simulink model "Q_2_1_4_PID_FF_Comp_Emulation_DISCRETE"  (R2024b)
settings: Solver=ode45  StartTime=0.0  StopTime=10  FixedStep=0.001  RelTol=1e-3
values from neighbouring files (symbols this model uses):
  B_eq = 6.6699e-7    (= 6.6699e-07)    [PID_calculations.m]    (also in Q1_2.2.1_Direct_digital_design.m; Q_2_2_1_Direct_digital_design.m; SS_Calculations.m; plant_calculations.m)
  delta_c = 1 / sqrt(2)    [PID_calculations.m]    (also in SS_Calculations.m; plant_calculations.m)
  J_eq = 6.0087e-7    (= 6.0087e-07)    [PID_calculations.m]    (also in Q1_2.2.1_Direct_digital_design.m; Q_2_2_1_Direct_digital_design.m; SS_Calculations.m; plant_calculations.m)
  K_D = K_P * T_D    [PID_calculations.m]
  K_I = K_P / T_I    [PID_calculations.m]
  K_P = DeltaK * cos(DeltaPhi)    [PID_calculations.m]
  K_W = 1 / T_W    (= 35.7142857143)    [PID_calculations.m]    (also in plant_calculations.m = 71.4285714286)
  kdrv = drv.dcgain    [PID_calculations.m]    (also in Q1_2.2.1_Direct_digital_design.m; Q_2_2_1_Direct_digital_design.m; SS_Calculations.m; plant_calculations.m)
  R_eq = mot.Ra + mot.Rs    [PID_calculations.m]    (also in Q1_2.2.1_Direct_digital_design.m; Q_2_2_1_Direct_digital_design.m; SS_Calculations.m; plant_calculations.m)
  T_DL = 1/ (2*w_gc)    [PID_calculations.m]    (also in discrete_time_basics.m)
  T_sample = 2e-3    (= 0.002)    [PID_calculations.m]    (also in discrete_time_basics.m = 0.001)
  tau_sf = 7.4967e-3    (= 0.0074967)    [PID_calculations.m]    (also in plant_calculations.m)
  w_c = 2 * pi * 20    (= 125.663706144)    [PID_calculations.m]    (also in SS_Calculations.m = 314.159265359; plant_calculations.m)
undefined symbols (not defined in the file or in its folder): DiscIntNeverNeededParam, dspblkCoreblockFVToolHelper, gbox, gcbh, mot, rads2rpm, rpm2rads, sens
settings Model: Creator=JS  LastModifiedBy=JS

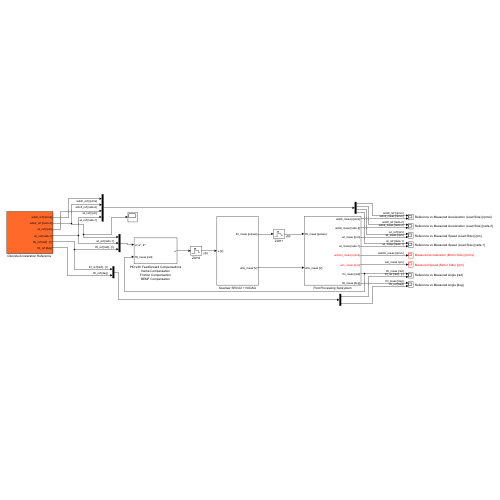
[thumbnail: Simulink's stored preview of the top-level diagram]
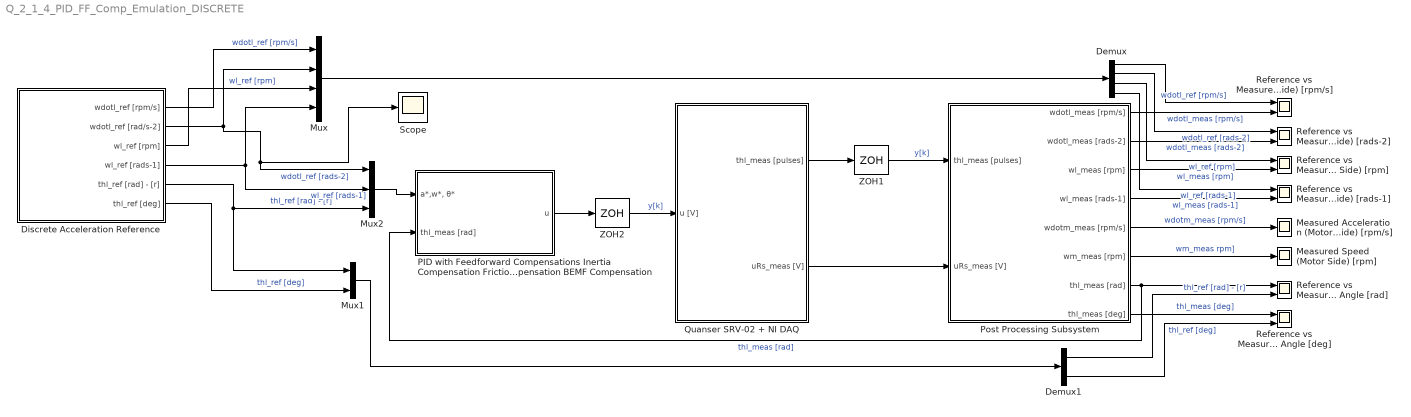
== system Q_2_1_4_PID_FF_Comp_Emulation_DISCRETE ==
  Demux : Demux
  Demux1 : Demux  Outputs=2
  "Discrete Acceleration Reference " : Subsystem
  Measured Acceleration (Motor Side) [rpm/s] : Scope
  Measured Speed (Motor Side) [rpm] : Scope
  Mux : Mux
  Mux1 : Mux  Inputs=2
  Mux2 : Mux  Inputs=3
  PID with Feedforward Compensations Inertia Compensation Friction Compensation BEMF Compensation : Subsystem
  Post Processing Subsystem : Subsystem
  Quanser SRV-02 + NI DAQ : Subsystem  mask(Quanser SRV-02 (with inertial load) + NI DAQ){Ts=0.001, fricType=Coulomb + viscous}
      mask prompts: Ts "NI DAQ Sample Time:"; fricType "Friction model"
      mask help: Quanser SRV-02 (with inertial load) + NI DAQ model.
      mask init:
      | %%  Sensors data
      | 
      | %   shunt resistor
      | sens.curr.Rs = 0.5;                         %   resistance [Ohm]   
      | sens.curr.uRs_std = 0.01;                   %   voltage noise standard dev [V]                           
      | sens.curr.uRs_var = sens.curr.uRs_std^2;	%   voltage noise variance [V^2]
      | 
      | %   Hewlett-Packard HEDS-5540#A06 optical encoder
      | sens.enc.ppr = 500*4;                       %   pulses per rotation
      | sens.enc.pulse2deg = 360/sens.enc.ppr;      %   [pulses] -> [deg]
      | sens.enc.pulse2rad = 2*pi/sens.enc.ppr;     %   [pulses] -> [rad]
      | sens.enc.deg2pulse = sens.enc.ppr/360;      %   [deg] -> [pulses]
      | sens.enc.rad2pulse = sens.enc.ppr/2/pi;     %   [rad] -> [pulses]
      | 
      | 
      | %%  Data acquisition board (daq) data
      | 
      | %   NI PCI-6221 DAC data
      | daq.dac.bits = 16;                                  %   resolution (bits)
      | daq.dac.fs   = 10;                                  %   full scale 
      | daq.dac.q    = 2*daq.dac.fs/(2^daq.dac.bits-1);     %	quantization
      | 
      | %   NI PCI-6221 ADC data
      | daq.adc.bits = 16;                                  %   resolution (bits)
      | daq.adc.fs   = 10;                                  %   full scale (as set in SLDRT Analog Input block)
      | daq.adc.q    = 2*daq.adc.fs/(2^daq.adc.bits-1);     %   quantization
      mask Help:
      | Riccardo Antonello (antonello@dei.unipd.it)
      | 
      | April 24, 2020
      | 
      | Dept. of Information Engineering, University of Padova
      mask TypeOptions fricType: Coulomb + viscous | Karnopp
  Reference vs Measured Acceleration (Load Side) [rads-2] : Scope  NumInputPorts=2
  Reference vs Measured Acceleration (Load Side) [rpm/s] : Scope  NumInputPorts=2
  "Reference vs Measured Angle [deg] " : Scope  NumInputPorts=2
  "Reference vs Measured Angle [rad] " : Scope  NumInputPorts=2
  Reference vs Measured Speed (Load Side) [rads-1] : Scope  NumInputPorts=2
  Reference vs Measured Speed (Load Side) [rpm] : Scope  NumInputPorts=2
  Scope : Scope
  ZOH1 : ZeroOrderHold  SampleTime=T_sample
  ZOH2 : ZeroOrderHold  SampleTime=T_sample
  wires:
  "Discrete Acceleration Reference "/5(thl_ref [rad] - [r]) -> Mux1/1, Mux2/3  "thl_ref [rad] - [r]"
  "Discrete Acceleration Reference "/2(wdotl_ref [rad/s-2]) -> Scope/1, Mux2/1, Mux/2  "wdotl_ref [rads-2]"
  "Discrete Acceleration Reference "/1(wdotl_ref [rpm/s]) -> Mux/1  "wdotl_ref [rpm/s]"
  "Discrete Acceleration Reference "/6(thl_ref [deg]) -> Mux1/2  "thl_ref [deg]"
  Quanser SRV-02 + NI DAQ/1(thl_meas [pulses]) -> ZOH1/1
  Quanser SRV-02 + NI DAQ/2(uRs_meas [V]) -> Post Processing Subsystem/2(uRs_meas [V])
  Post Processing Subsystem/1(wdotl_meas [rpm/s]) -> Reference vs Measured Acceleration (Load Side) [rpm/s]/2  "wdotl_meas [rpm/s]"
  Post Processing Subsystem/8(thl_meas [deg]) -> "Reference vs Measured Angle [deg] "/1  "thl_meas [deg]"
  Post Processing Subsystem/7(thl_meas [rad]) -> "Reference vs Measured Angle [rad] "/1, PID with Feedforward Compensations Inertia Compensation Friction Compensation BEMF Compensation/2(thl_meas [rad])  "thl_meas [rad]"
  Post Processing Subsystem/2(wdotl_meas [rads-2]) -> Reference vs Measured Acceleration (Load Side) [rads-2]/2  "wdotl_meas [rads-2]"
  Post Processing Subsystem/5(wdotm_meas [rpm/s]) -> Measured Acceleration (Motor Side) [rpm/s]/1  "wdotm_meas [rpm/s]"
  Post Processing Subsystem/6(wm_meas [rpm]) -> Measured Speed (Motor Side) [rpm]/1  "wm_meas rpm]"
  Post Processing Subsystem/4(wl_meas [rads-1]) -> Reference vs Measured Speed (Load Side) [rads-1]/2  "wl_meas [rads-1]"
  Post Processing Subsystem/3(wl_meas [rpm]) -> Reference vs Measured Speed (Load Side) [rpm]/2  "wl_meas [rpm]"
  "Discrete Acceleration Reference "/3(wl_ref [rpm]) -> Mux/3  "wl_ref [rpm]"
  "Discrete Acceleration Reference "/4(wl_ref [rads-1]) -> Mux2/2, Mux/4  "wl_ref [rads-1]"
  Demux/1 -> Reference vs Measured Acceleration (Load Side) [rpm/s]/1  "wdotl_ref [rpm/s]"
  Demux/2 -> Reference vs Measured Acceleration (Load Side) [rads-2]/1  "wdotl_ref [rads-2]"
  Demux/3 -> Reference vs Measured Speed (Load Side) [rpm]/1  "wl_ref [rpm]"
  Demux/4 -> Reference vs Measured Speed (Load Side) [rads-1]/1  "wl_ref [rads-1]"
  Mux/1 -> Demux/1
  Mux1/1 -> Demux1/1
  Demux1/1 -> "Reference vs Measured Angle [rad] "/2  "thl_ref [rad] - [r]"
  Demux1/2 -> "Reference vs Measured Angle [deg] "/2  "thl_ref [deg]"
  PID with Feedforward Compensations Inertia Compensation Friction Compensation BEMF Compensation/1(u) -> ZOH2/1
  Mux2/1 -> PID with Feedforward Compensations Inertia Compensation Friction Compensation BEMF Compensation/1("a*,w*, θ*")
  ZOH1/1 -> Post Processing Subsystem/1(thl_meas [pulses])  "y[k]"
  ZOH2/1 -> Quanser SRV-02 + NI DAQ/1(u [V])  "y[k]"

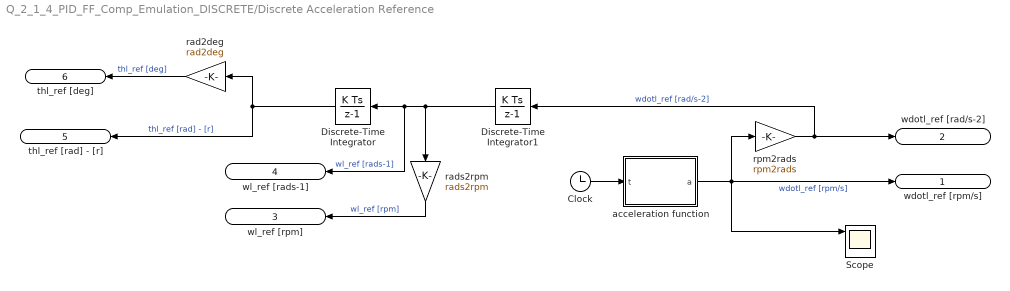
== system Q_2_1_4_PID_FF_Comp_Emulation_DISCRETE/Discrete Acceleration Reference  ==
  Clock : Clock
  Discrete-Time Integrator : DiscreteIntegrator  gainval=K_sample  SampleTime=T_sample  ICPrevOutput=DiscIntNeverNeededParam  ICPrevScaledInput=DiscIntNeverNeededParam
  Discrete-Time Integrator1 : DiscreteIntegrator  gainval=K_sample  SampleTime=T_sample  ICPrevOutput=DiscIntNeverNeededParam  ICPrevScaledInput=DiscIntNeverNeededParam
  Scope : Scope  NumInputPorts=3
  acceleration function : MATLAB Function  TreatAsAtomicUnit=on
  rad2deg : Gain  Gain=rad2deg
  rads2rpm : Gain  Gain=rads2rpm
  rpm2rads : Gain  Gain=rpm2rads
  wdotl_ref [rpm/s] : Outport
  wdotl_ref [rad/s-2] : Outport  Port=2
  wl_ref [rpm] : Outport  Port=3
  wl_ref [rads-1] : Outport  Port=4
  thl_ref [rad] - [r] : Outport  Port=5
  thl_ref [deg] : Outport  Port=6
  wires:
  Discrete-Time Integrator/1 -> thl_ref [rad] - [r]/1, rad2deg/1  "thl_ref [rad] - [r]"
  acceleration function/1(a) -> Scope/1, rpm2rads/1, wdotl_ref [rpm/s]/1  "wdotl_ref [rpm/s]"
  Discrete-Time Integrator1/1 -> Discrete-Time Integrator/1, wl_ref [rads-1]/1, rads2rpm/1  "wl_ref [rads-1]"
  rads2rpm/1 -> wl_ref [rpm]/1  "wl_ref [rpm]"
  Clock/1 -> acceleration function/1(t)
  rpm2rads/1 -> Discrete-Time Integrator1/1, wdotl_ref [rad/s-2]/1  "wdotl_ref [rad/s-2]"
  rad2deg/1 -> thl_ref [deg]/1  "thl_ref [deg]"

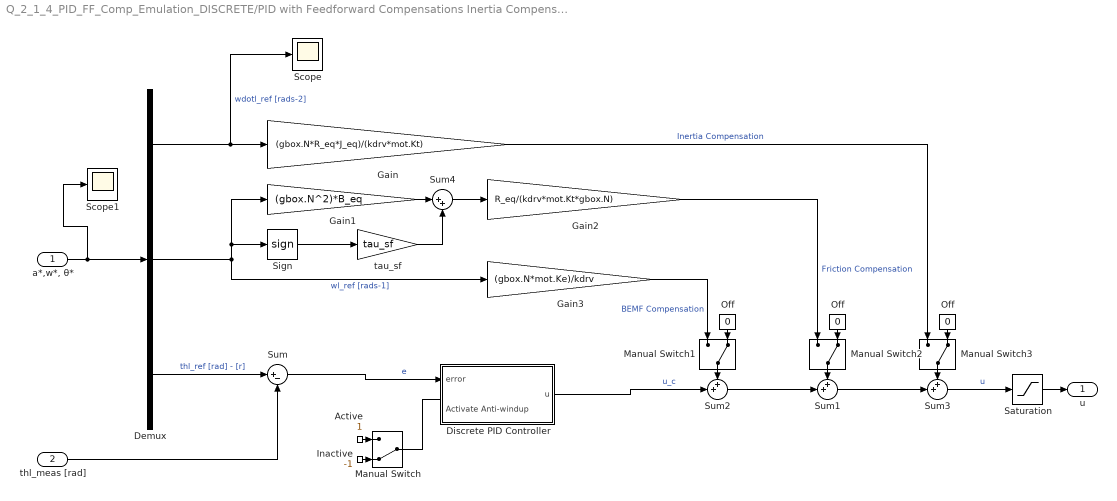
== system Q_2_1_4_PID_FF_Comp_Emulation_DISCRETE/PID with Feedforward Compensations Inertia Compensation Friction Compensation BEMF Compensation ==
  "a*,w*, θ*" : Inport
  thl_meas [rad] : Inport  Port=2
  Active : Constant
  Demux : Demux  Outputs=3
  Discrete PID Controller : Subsystem
  Gain : Gain  Gain=(gbox.N*R_eq*J_eq)/(kdrv*mot.Kt)
  Gain1 : Gain  Gain=(gbox.N^2)*B_eq
  Gain2 : Gain  Gain=R_eq/(kdrv*mot.Kt*gbox.N)
  Gain3 : Gain  Gain=(gbox.N*mot.Ke)/kdrv
  Inactive : Constant  Value=-1
  Manual Switch{,1..3} (4 alike) : ManualSwitch  CurrentSetting=0
  Off : Constant  Value=0
  "Off " : Constant  Value=0
  "Off  " : Constant  Value=0
  Saturation : Saturate  UpperLimit=10  LowerLimit=-10
  Scope : Scope
  Scope1 : Scope
  Sign : Signum
  Sum : Sum  Inputs=|+-
  Sum1 : Sum  Inputs=++|
  Sum2 : Sum  Inputs=++|
  Sum3 : Sum  Inputs=++|
  Sum4 : Sum  Inputs=|++
  tau_sf : Gain  Gain=tau_sf
  u : Outport
  wires:
  "a*,w*, θ*"/1 -> Scope1/1, Demux/1
  thl_meas [rad]/1 -> Sum/2
  Sum/1 -> Discrete PID Controller/1(error)  "e"
  Sum3/1 -> Saturation/1  "u"
  Sum1/1 -> Sum3/2
  Sum2/1 -> Sum1/2
  Discrete PID Controller/1(u) -> Sum2/2  "u_c"
  Demux/1 -> Scope/1, Gain/1  "wdotl_ref [rads-2]"
  Demux/2 -> Sign/1, Gain1/1, Gain3/1  "wl_ref [rads-1]"
  Demux/3 -> Sum/1  "thl_ref [rad] - [r]"
  Gain/1 -> Manual Switch3/1  "Inertia Compensation"
  Gain1/1 -> Sum4/1
  tau_sf/1 -> Sum4/2
  Sum4/1 -> Gain2/1
  Gain2/1 -> Manual Switch2/1  "Friction Compensation"
  Gain3/1 -> Manual Switch1/1  "BEMF Compensation"
  Saturation/1 -> u/1
  Sign/1 -> tau_sf/1
  Inactive/1 -> Manual Switch/2
  Active/1 -> Manual Switch/1
  Manual Switch/1 -> ?
  Off/1 -> Manual Switch1/2
  Manual Switch1/1 -> Sum2/1
  "Off "/1 -> Manual Switch2/2
  Manual Switch2/1 -> Sum1/1
  Manual Switch3/1 -> Sum3/1
  "Off  "/1 -> Manual Switch3/2

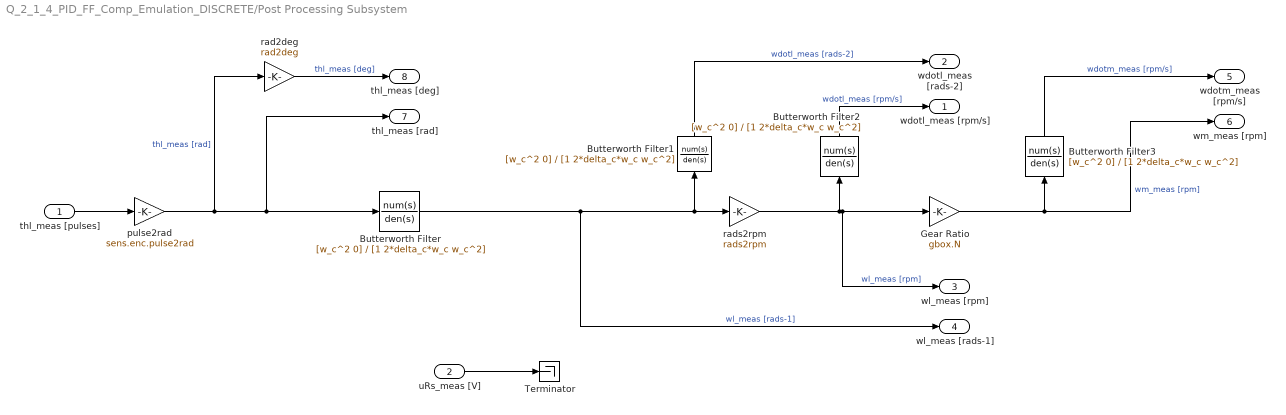
== system Q_2_1_4_PID_FF_Comp_Emulation_DISCRETE/Post Processing Subsystem ==
  thl_meas [pulses] : Inport
  uRs_meas [V] : Inport  Port=2
  Butterworth Filter{,1..3} (4 alike) : TransferFcn  Numerator=[w_c^2 0]  Denominator=[1 2*delta_c*w_c w_c^2]
  Gear Ratio : Gain  Gain=gbox.N
  Terminator : Terminator
  pulse2rad : Gain  Gain=sens.enc.pulse2rad
  rad2deg : Gain  Gain=rad2deg
  rads2rpm : Gain  Gain=rads2rpm
  wdotl_meas [rpm/s] : Outport
  wdotl_meas [rads-2] : Outport  Port=2
  wl_meas [rpm] : Outport  Port=3
  wl_meas [rads-1] : Outport  Port=4
  wdotm_meas [rpm/s] : Outport  Port=5
  wm_meas [rpm] : Outport  Port=6
  thl_meas [rad] : Outport  Port=7
  thl_meas [deg] : Outport  Port=8
  wires:
  pulse2rad/1 -> Butterworth Filter/1, thl_meas [rad]/1, rad2deg/1  "thl_meas [rad]"
  rad2deg/1 -> thl_meas [deg]/1  "thl_meas [deg]"
  uRs_meas [V]/1 -> Terminator/1
  thl_meas [pulses]/1 -> pulse2rad/1
  Butterworth Filter3/1 -> wdotm_meas [rpm/s]/1  "wdotm_meas [rpm/s]"
  Butterworth Filter2/1 -> wdotl_meas [rpm/s]/1  "wdotl_meas [rpm/s]"
  rads2rpm/1 -> Gear Ratio/1, wl_meas [rpm]/1, Butterworth Filter2/1  "wl_meas [rpm]"
  Butterworth Filter1/1 -> wdotl_meas [rads-2]/1  "wdotl_meas [rads-2]"
  Gear Ratio/1 -> wm_meas [rpm]/1, Butterworth Filter3/1  "wm_meas [rpm]"
  Butterworth Filter/1 -> Butterworth Filter1/1, rads2rpm/1, wl_meas [rads-1]/1  "wl_meas [rads-1]"

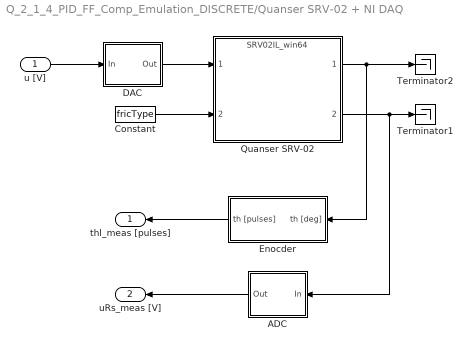
== system Q_2_1_4_PID_FF_Comp_Emulation_DISCRETE/Quanser SRV-02 + NI DAQ ==
  u [V] : Inport
  ADC : Subsystem
  Constant : Constant  Value=fricType
  DAC : Subsystem
  Enocder : Subsystem
  Quanser SRV-02 : ModelReference  ModelNameDialog=SRV02IL_win64.slxp  ModelReferenceVersion=1.44  CopyOfModelProtected=on
  Terminator1 : Terminator
  Terminator2 : Terminator
  thl_meas [pulses] : Outport
  uRs_meas [V] : Outport  Port=2
  wires:
  Enocder/1(th [pulses]) -> thl_meas [pulses]/1
  ADC/1(Out) -> uRs_meas [V]/1
  DAC/1(Out) -> Quanser SRV-02/1
  Quanser SRV-02/2 -> ADC/1(In), Terminator1/1
  u [V]/1 -> DAC/1(In)
  Quanser SRV-02/1 -> Enocder/1(th [deg]), Terminator2/1
  Constant/1 -> Quanser SRV-02/2

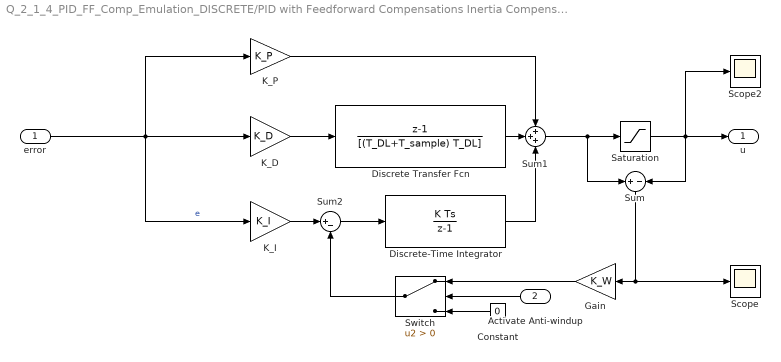
== system Q_2_1_4_PID_FF_Comp_Emulation_DISCRETE/PID with Feedforward Compensations Inertia Compensation Friction Compensation BEMF Compensation/Discrete PID Controller ==
  error : Inport
  Activate Anti-windup : Inport  Port=2
  Constant : Constant  Value=0
  Discrete Transfer Fcn : DiscreteTransferFcn  LoadFcn=dspblkCoreblockFVToolHelper(gcbh,'load');  Numerator=[1 -1]  Denominator=[(T_DL+T_sample) T_DL]
      settings: CopyFcn=dspblkCoreblockFVToolHelper(gcbh,'copy');  DeleteFcn=dspblkCoreblockFVToolHelper(gcbh,'close');  ModelCloseFcn=dspblkCoreblockFVToolHelper(gcbh,'close');  PreSaveFcn=dspblkCoreblockFVToolHelper(gcbh,'presave');  PostSaveFcn=dspblkCoreblockFVToolHelper(gcbh,'postsave');  CloseFcn=dspblkCoreblockFVToolHelper(gcbh,'close');
  Discrete-Time Integrator : DiscreteIntegrator  gainval=K_sample  SampleTime=T_sample  ICPrevOutput=DiscIntNeverNeededParam  ICPrevScaledInput=DiscIntNeverNeededParam
  Gain : Gain  Gain=K_W
  K_D : Gain  Gain=K_D
  K_I : Gain  Gain=K_I
  K_P : Gain  Gain=K_P
  Saturation : Saturate  UpperLimit=10  LowerLimit=-10  LinearizeAsGain=off
  Scope : Scope
  Scope2 : Scope
  Sum : Sum  Inputs=+|-
  Sum1 : Sum  Inputs=+++
  Sum2 : Sum  Inputs=|+-
  Switch : Switch  Criteria=u2 > Threshold  SaturateOnIntegerOverflow=off  InputSameDT=off
  u : Outport
  wires:
  Sum1/1 -> Saturation/1, Sum/1
  Saturation/1 -> Scope2/1, u/1, Sum/2
  Gain/1 -> Switch/1
  error/1 -> K_P/1, K_I/1, K_D/1  "e"
  Activate Anti-windup/1 -> Switch/2
  Constant/1 -> Switch/3
  Sum/1 -> Scope/1, Gain/1
  Switch/1 -> Sum2/2
  Discrete-Time Integrator/1 -> Sum1/3
  K_I/1 -> Sum2/1
  Sum2/1 -> Discrete-Time Integrator/1
  Discrete Transfer Fcn/1 -> Sum1/2
  K_D/1 -> Discrete Transfer Fcn/1
  K_P/1 -> Sum1/1

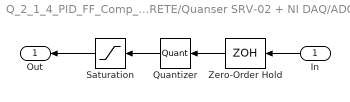
== system Q_2_1_4_PID_FF_Comp_Emulation_DISCRETE/Quanser SRV-02 + NI DAQ/ADC ==
  In : Inport
  Quantizer : Quantizer  QuantizationInterval=daq.adc.q
  Saturation : Saturate  UpperLimit=daq.adc.fs  LowerLimit=-daq.adc.fs
  Zero-Order Hold : ZeroOrderHold  SampleTime=Ts
  Out : Outport
  wires:
  Saturation/1 -> Out/1
  In/1 -> Zero-Order Hold/1
  Quantizer/1 -> Saturation/1
  Zero-Order Hold/1 -> Quantizer/1

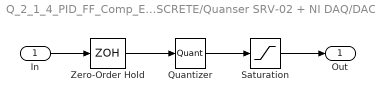
== system Q_2_1_4_PID_FF_Comp_Emulation_DISCRETE/Quanser SRV-02 + NI DAQ/DAC ==
  In : Inport
  Quantizer : Quantizer  QuantizationInterval=daq.dac.q
  Saturation : Saturate  UpperLimit=daq.dac.fs  LowerLimit=-daq.dac.fs
  Zero-Order Hold : ZeroOrderHold  SampleTime=Ts
  Out : Outport
  wires:
  Quantizer/1 -> Saturation/1
  In/1 -> Zero-Order Hold/1
  Zero-Order Hold/1 -> Quantizer/1
  Saturation/1 -> Out/1

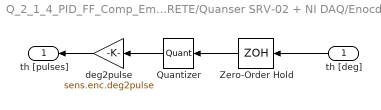
== system Q_2_1_4_PID_FF_Comp_Emulation_DISCRETE/Quanser SRV-02 + NI DAQ/Enocder ==
  th [deg] : Inport
  Quantizer : Quantizer  QuantizationInterval=sens.enc.pulse2deg
  Zero-Order Hold : ZeroOrderHold  SampleTime=Ts
  deg2pulse : Gain  Gain=sens.enc.deg2pulse
  th [pulses] : Outport
  wires:
  Quantizer/1 -> deg2pulse/1
  th [deg]/1 -> Zero-Order Hold/1
  Zero-Order Hold/1 -> Quantizer/1
  deg2pulse/1 -> th [pulses]/1

== matlab function Q_2_1_4_PID_FF_Comp_Emulation_DISCRETE/Discrete Acceleration Reference /acceleration function ==
  data: t input; a output
function a = a_star_i(t)

t_mod = mod(t, 3);
a = zeros(size(t));

a(t_mod >= 0   & t_mod < 0.5)  =  900;
a(t_mod >= 0.5 & t_mod < 1)    =    0;
a(t_mod >= 1   & t_mod < 2)    = -900;
a(t_mod >= 2   & t_mod < 2.5)  =    0;
a(t_mod >= 2.5 & t_mod < 3)    =  900;
end
